simulink model "Linear_MPC_design_test"  (R2024a)
settings: Solver=VariableStepAuto  StartTime=0.0  StopTime=5  MaxStep=0.1  RelTol=1e-3
model workspace (MAT data in the model file):
  Sig = Simulink.Signal
  Sig.DataType = 'auto'
  Sig.Dimensions = -1
  Sig.DimensionsMode = 'auto'
  Sig.Complexity = 'auto'
  Sig.SampleTime = -1
  Sig.SamplingMode = 'auto'
undefined symbols (not defined in the file): reference, Ts
libraries: Bonus_Library x2, cstblocks x1, mpclib x1
settings Model: PauseTimes=4  Creator=mulusoy  LastModifiedBy=User
settings OptimizationCC: ReuseModelBlockBuffer=off
settings RTWCC: GPUComputeCapability=3.5

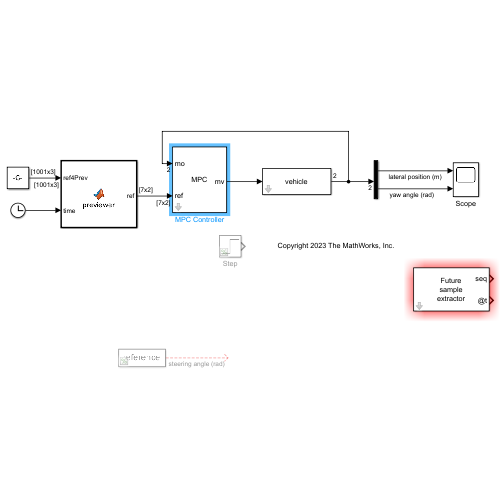
[thumbnail: Simulink's stored preview of the top-level diagram]
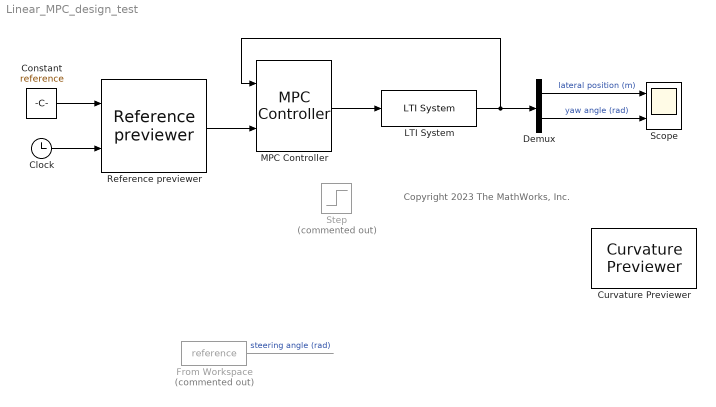
== system Linear_MPC_design_test ==
  note: Copyright 2023 The MathWorks, Inc.
  Clock : Clock
  Constant : Constant  Value=reference
  Curvature Previewer : Bonus_Library/Curvature Previewer  signal=md  ts=.001  steps=10000
  Demux : Demux  Outputs=2
  From Workspace : FromWorkspace  Commented=on  VariableName=reference
  LTI System : cstblocks/LTI System  sys=vehicle  IC=[]  PadeOrder=0
  MPC Controller : mpclib/MPC Controller  SCDEnableBlockLinearizationSpecification=on  is_multiple=0  enable_value=0  return_u0=off  updateMPCinCallerWorkspace=on  md_inport=off  mv_inport=off  uref_inport=off  return_cost=off  return_mvseq=off  return_qpstatus=off  return_xseq=off  return_state=off  return_ovseq=off  state_inport=off  umin_inport=off  umax_inport=off  ymin_inport=off  ymax_inport=off  cc_inport=off  ywt_inport=off  uwt_inport=off  duwt_inport=off  rhoeps_inport=off  pm_inport=off  MaximumP=10  HorizonChoice=FixedHorizon  n_ts=1  n_p=10  n_mv=1  n_md=1  n_ud=0  n_mo=2  n_uo=0  BlockDataType=double  SampleTimeInherited=off  switch_inport=off
  Reference previewer : Bonus_Library/Reference previewer  SystemSampleTime=Ts  VariantActivationTime=update diagram  AllowFlexibleInterface=on  Latency=0  AutoFrameSizeCalculation=off
  Scope : Scope  NumInputPorts=2
  Step : Step  Commented=on  Time=4  After=pi/6  SampleTime=0
  wires:
  LTI System/1 -> MPC Controller/1, Demux/1
  Demux/1 -> Scope/1  "lateral position (m)"
  Demux/2 -> Scope/2  "yaw angle (rad)"
  From Workspace/1 -> ?  "steering angle (rad)"
  MPC Controller/1 -> LTI System/1
  Reference previewer/1 -> MPC Controller/2
  Clock/1 -> Reference previewer/2
  Constant/1 -> Reference previewer/1
